simulink model "CellTemp"  (R2017b)
settings: Solver=VariableStepAuto  StartTime=0.0  StopTime=10.0  RelTol=1e-3
undefined symbols (not defined in the file): Battery, Brake, DriveCycle, Driver, g, magnitude, Motor, Sim, TorqueController, TrqSplit, Veh
libraries: simulink x2, AMKMotor x1
settings Model: Creator=Harjot  LastModifiedBy=Harjot

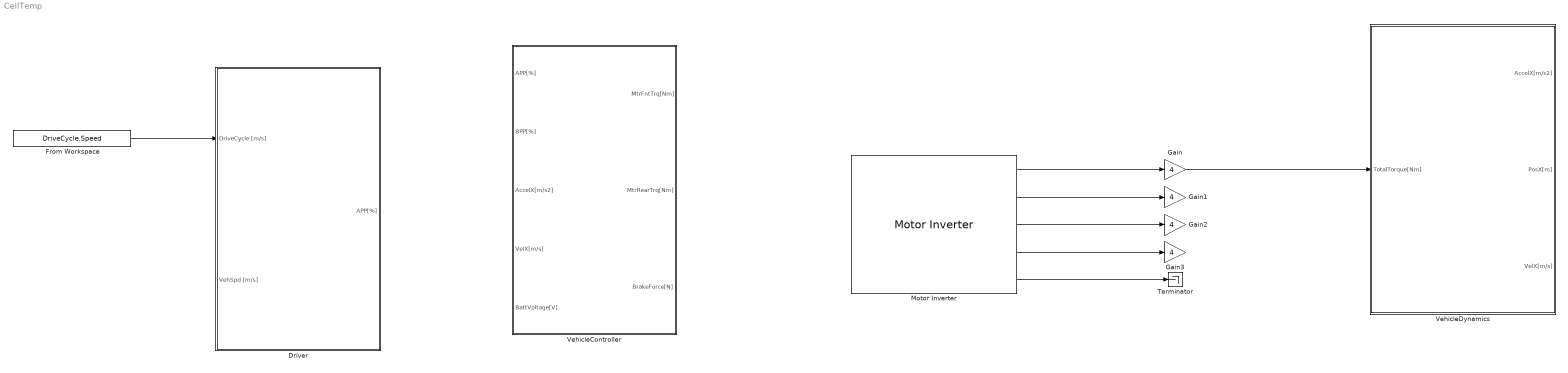
== system CellTemp ==
  Driver : Subsystem
  From Workspace : FromWorkspace  VariableName=DriveCycle.Speed  SampleTime=0
  Gain{,1..3} (4 alike) : Gain  Gain=4
  Motor Inverter : AMKMotor/Motor Inverter
  Terminator : Terminator
  VehicleController : Subsystem  VariantControl=CSMode == 1
  VehicleDynamics : Subsystem
  wires:
  Motor Inverter/1 -> Gain/1
  Gain/1 -> VehicleDynamics/1(TotalTorque[Nm])
  Motor Inverter/2 -> Gain1/1
  Motor Inverter/3 -> Gain2/1
  Motor Inverter/4 -> Gain3/1
  Motor Inverter/5 -> Terminator/1
  From Workspace/1 -> Driver/1(DriveCycle [m/s])

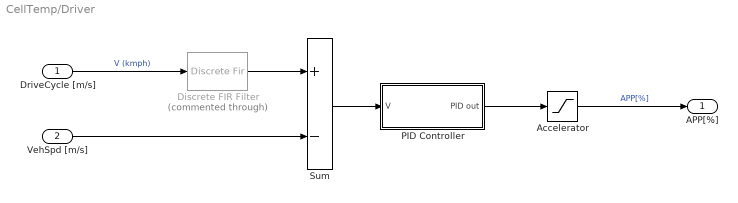
== system CellTemp/Driver ==
  DriveCycle [m/s] : Inport
  VehSpd [m/s] : Inport  Port=2
  Accelerator : Saturate  UpperLimit=100  LowerLimit=0
  Discrete FIR Filter : DiscreteFir  Commented=through  Coefficients=[100:-1:0]/sum([100:-1:0])  SampleTime=Sim.TimeStep
  PID Controller : Subsystem
  Sum : Sum  Inputs=+-
  APP[%] : Outport
  wires:
  VehSpd [m/s]/1 -> Sum/2
  Sum/1 -> PID Controller/1(V)
  DriveCycle [m/s]/1 -> Discrete FIR Filter/1  "V (kmph)"
  PID Controller/1("PID out ") -> Accelerator/1
  Accelerator/1 -> APP[%]/1  "APP[%]"
  Discrete FIR Filter/1 -> Sum/1

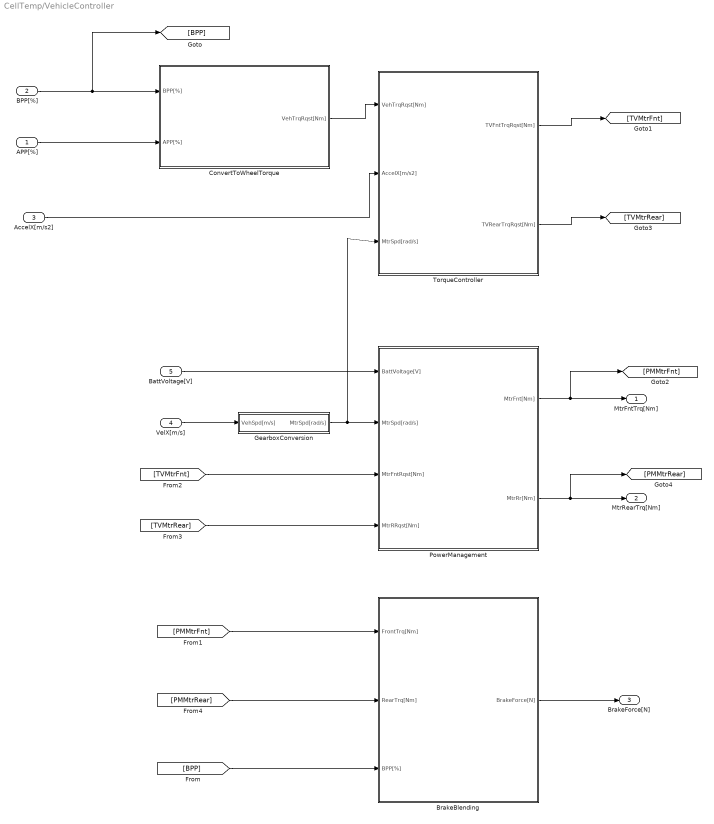
== system CellTemp/VehicleController ==
  APP[%] : Inport
  BPP[%] : Inport  Port=2
  AccelX[m/s2] : Inport  Port=3
  VelX[m/s] : Inport  Port=4
  BattVoltage[V] : Inport  Port=5
  BrakeBlending : Subsystem
  ConvertToWheelTorque : Subsystem
  GearboxConversion : Subsystem
  PowerManagement : Subsystem
  TorqueController : Subsystem
  MtrFntTrq[Nm] : Outport
  MtrRearTrq[Nm] : Outport  Port=2
  BrakeForce[N] : Outport  Port=3
  wires:
  APP[%]/1 -> ConvertToWheelTorque/2(APP[%])
  BPP[%]/1 -> ConvertToWheelTorque/1(BPP[%]), [BPP]
  [PMMtrRear] -> BrakeBlending/2(RearTrq[Nm])
  [PMMtrFnt] -> BrakeBlending/1(FrontTrq[Nm])
  [BPP] -> BrakeBlending/3(BPP[%])
  BrakeBlending/1(BrakeForce[N]) -> BrakeForce[N]/1
  ConvertToWheelTorque/1(VehTrqRqst[Nm]) -> TorqueController/1(VehTrqRqst[Nm])
  GearboxConversion/1(MtrSpd[rad/s]) -> TorqueController/3(MtrSpd[rad/s]), PowerManagement/2(MtrSpd[rad/s])
  VelX[m/s]/1 -> GearboxConversion/1(VehSpd[m/s])
  PowerManagement/2(MtrRr[Nm]) -> MtrRearTrq[Nm]/1, [PMMtrRear]
  PowerManagement/1(MtrFnt[Nm]) -> MtrFntTrq[Nm]/1, [PMMtrFnt]
  [TVMtrRear] -> PowerManagement/4(MtrRRqst[Nm])
  [TVMtrFnt] -> PowerManagement/3(MtrFntRqst[Nm])
  BattVoltage[V]/1 -> PowerManagement/1(BattVoltage[V])
  TorqueController/2(TVRearTrqRqst[Nm]) -> [TVMtrRear]
  TorqueController/1(TVFntTrqRqst[Nm]) -> [TVMtrFnt]
  AccelX[m/s2]/1 -> TorqueController/2(AccelX[m/s2])

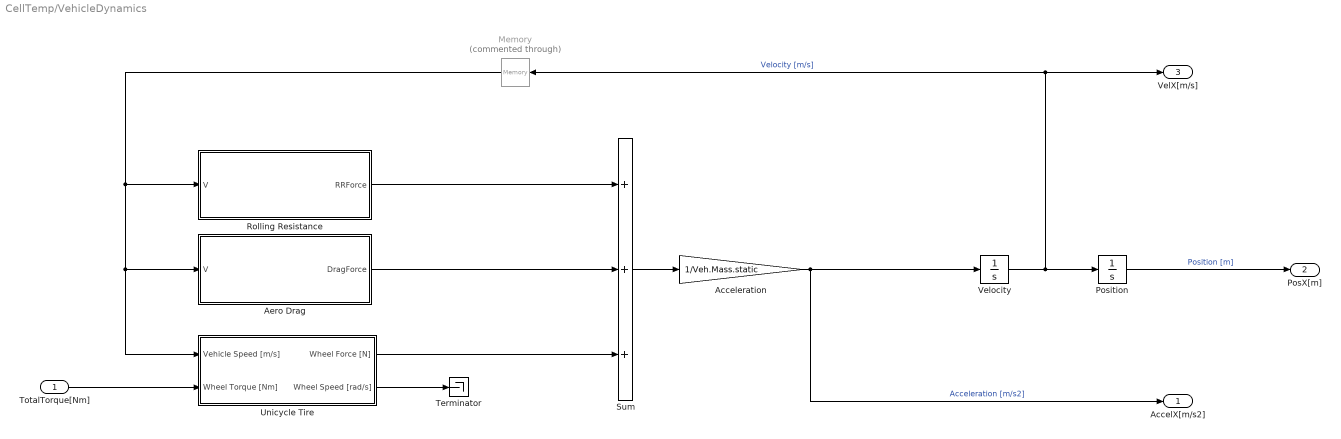
== system CellTemp/VehicleDynamics ==
  TotalTorque[Nm] : Inport
  Acceleration : Gain  Gain=1/Veh.Mass.static
  Aero Drag : Subsystem
  Memory : Memory  Commented=through
  Position : Integrator
  Rolling Resistance : Subsystem
  Sum : Sum  Inputs=+++
  Terminator : Terminator
  Unicycle Tire : Subsystem
  Velocity : Integrator  InitialCondition=DriveCycle.Vi
  AccelX[m/s2] : Outport
  PosX[m] : Outport  Port=2
  VelX[m/s] : Outport  Port=3
  wires:
  Memory/1 -> Unicycle Tire/1(Vehicle Speed [m/s]), Aero Drag/1(V), Rolling Resistance/1(V)
  Acceleration/1 -> AccelX[m/s2]/1, Velocity/1  "Acceleration [m/s2]"
  TotalTorque[Nm]/1 -> Unicycle Tire/2(Wheel Torque [Nm])
  Rolling Resistance/1(RRForce) -> Sum/1
  Aero Drag/1(DragForce) -> Sum/2
  Sum/1 -> Acceleration/1
  Unicycle Tire/1(Wheel Force [N]) -> Sum/3
  Unicycle Tire/2(Wheel Speed [rad/s]) -> Terminator/1
  Velocity/1 -> Memory/1, VelX[m/s]/1, Position/1  "Velocity [m/s]"
  Position/1 -> PosX[m]/1  "Position [m]"

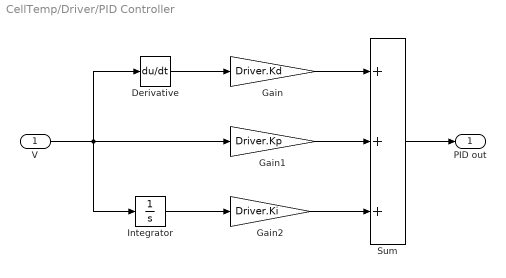
== system CellTemp/Driver/PID Controller ==
  V : Inport
  Derivative : Derivative
  Gain : Gain  Gain=Driver.Kd
  Gain1 : Gain  Gain=Driver.Kp
  Gain2 : Gain  Gain=Driver.Ki
  Integrator : Integrator
  Sum : Sum  Inputs=+++
  "PID out " : Outport
  wires:
  Integrator/1 -> Gain2/1
  V/1 -> Integrator/1, Derivative/1, Gain1/1
  Gain/1 -> Sum/1
  Gain1/1 -> Sum/2
  Gain2/1 -> Sum/3
  Sum/1 -> "PID out "/1
  Derivative/1 -> Gain/1

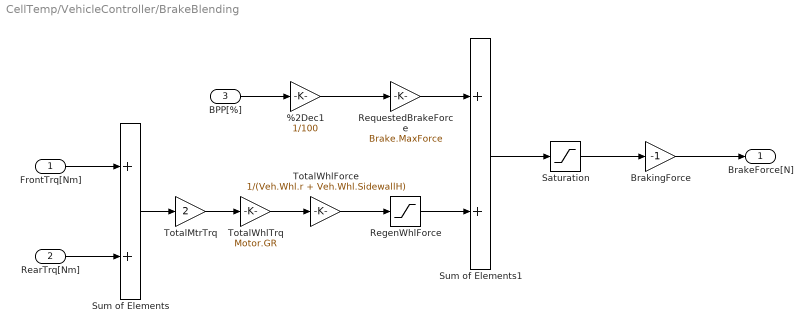
== system CellTemp/VehicleController/BrakeBlending ==
  FrontTrq[Nm] : Inport
  RearTrq[Nm] : Inport  Port=2
  BPP[%] : Inport  Port=3
  %2Dec1 : Gain  Gain=1/100
  BrakingForce : Gain  Gain=-1
  RegenWhlForce : Saturate  UpperLimit=0  LowerLimit=-inf
  RequestedBrakeForce : Gain  Gain=Brake.MaxForce
  Saturation : Saturate  UpperLimit=inf  LowerLimit=0
  Sum of Elements : Sum  Inputs=2
  Sum of Elements1 : Sum
  TotalMtrTrq : Gain  Gain=2
  TotalWhlForce : Gain  Gain=1/(Veh.Whl.r + Veh.Whl.SidewallH)
  TotalWhlTrq : Gain  Gain=Motor.GR
  BrakeForce[N] : Outport
  wires:
  BrakingForce/1 -> BrakeForce[N]/1
  RegenWhlForce/1 -> Sum of Elements1/2
  TotalWhlTrq/1 -> TotalWhlForce/1
  Sum of Elements/1 -> TotalMtrTrq/1
  Saturation/1 -> BrakingForce/1
  Sum of Elements1/1 -> Saturation/1
  TotalWhlForce/1 -> RegenWhlForce/1
  RequestedBrakeForce/1 -> Sum of Elements1/1
  BPP[%]/1 -> %2Dec1/1
  %2Dec1/1 -> RequestedBrakeForce/1
  TotalMtrTrq/1 -> TotalWhlTrq/1
  RearTrq[Nm]/1 -> Sum of Elements/2
  FrontTrq[Nm]/1 -> Sum of Elements/1

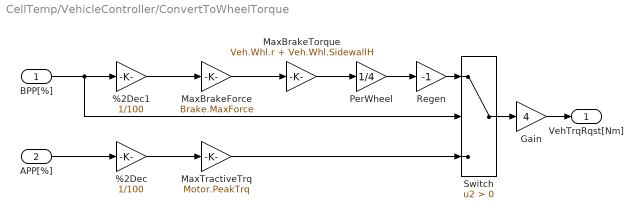
== system CellTemp/VehicleController/ConvertToWheelTorque ==
  BPP[%] : Inport
  APP[%] : Inport  Port=2
  %2Dec : Gain  Gain=1/100
  %2Dec1 : Gain  Gain=1/100
  Gain : Gain  Gain=4
  MaxBrakeForce : Gain  Gain=Brake.MaxForce
  MaxBrakeTorque : Gain  Gain=Veh.Whl.r + Veh.Whl.SidewallH
  "MaxTractiveTrq " : Gain  Gain=Motor.PeakTrq
  PerWheel : Gain  Gain=1/4
  Regen : Gain  Gain=-1
  Switch : Switch  Criteria=u2 > Threshold
  VehTrqRqst[Nm] : Outport
  wires:
  Regen/1 -> Switch/1
  APP[%]/1 -> %2Dec/1
  Switch/1 -> Gain/1
  %2Dec1/1 -> MaxBrakeForce/1
  BPP[%]/1 -> %2Dec1/1, Switch/2
  MaxBrakeTorque/1 -> PerWheel/1
  MaxBrakeForce/1 -> MaxBrakeTorque/1
  %2Dec/1 -> "MaxTractiveTrq "/1
  "MaxTractiveTrq "/1 -> Switch/3
  PerWheel/1 -> Regen/1
  Gain/1 -> VehTrqRqst[Nm]/1

== system CellTemp/VehicleController/GearboxConversion ==
  VehSpd[m/s] : Inport
  MotorGR : Gain  Gain=Motor.GR
  WheelRadius : Gain  Gain=1/(Veh.Whl.r + Veh.Whl.SidewallH)
  MtrSpd[rad/s] : Outport
  wires:
  MotorGR/1 -> MtrSpd[rad/s]/1  "MtrSpd [rad/s]"
  VehSpd[m/s]/1 -> WheelRadius/1
  WheelRadius/1 -> MotorGR/1  "WhlSpd [rad/s]"

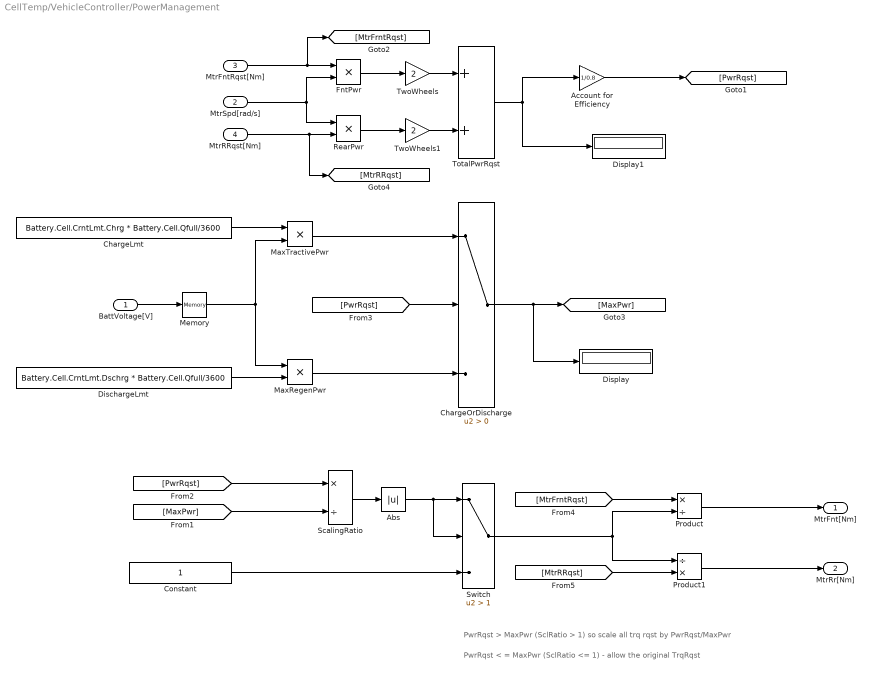
== system CellTemp/VehicleController/PowerManagement ==
  note: PwrRqst < = MaxPwr (SclRatio <= 1) - allow the original TrqRqst
  note: PwrRqst > MaxPwr (SclRatio > 1) so scale all trq rqst by PwrRqst/MaxPwr
  BattVoltage[V] : Inport
  MtrSpd[rad/s] : Inport  Port=2
  MtrFntRqst[Nm] : Inport  Port=3
  MtrRRqst[Nm] : Inport  Port=4
  Abs : Abs
  Account for Efficiency : Gain  Gain=1/0.8
  ChargeLmt : Constant  Value=Battery.Cell.CrntLmt.Chrg * Battery.Cell.Qfull/3600
  ChargeOrDischarge : Switch  Criteria=u2 > Threshold
  Constant : Constant
  DischargeLmt : Constant  Value=Battery.Cell.CrntLmt.Dschrg * Battery.Cell.Qfull/3600
  Display : Display
  Display1 : Display
  FntPwr : Product
  MaxRegenPwr : Product
  MaxTractivePwr : Product
  Memory : Memory  InitialCondition=600
  Product : Product  Inputs=*/
  Product1 : Product  Inputs=/*
  RearPwr : Product
  ScalingRatio : Product  Inputs=*/
  Switch : Switch  Criteria=u2 > Threshold  Threshold=1
  TotalPwrRqst : Sum
  TwoWheels : Gain  Gain=2
  TwoWheels1 : Gain  Gain=2
  MtrFnt[Nm] : Outport
  MtrRr[Nm] : Outport  Port=2
  wires:
  Memory/1 -> MaxRegenPwr/1, MaxTractivePwr/2
  Constant/1 -> Switch/3
  Product1/1 -> MtrRr[Nm]/1
  Product/1 -> MtrFnt[Nm]/1
  [MtrRRqst] -> Product1/2
  [MtrFrntRqst] -> Product/1
  Switch/1 -> Product1/1, Product/2
  MtrFntRqst[Nm]/1 -> FntPwr/1, [MtrFrntRqst]
  [PwrRqst] -> ChargeOrDischarge/2
  TwoWheels/1 -> TotalPwrRqst/1
  TotalPwrRqst/1 -> Account for Efficiency/1, Display1/1
  TwoWheels1/1 -> TotalPwrRqst/2
  RearPwr/1 -> TwoWheels1/1
  FntPwr/1 -> TwoWheels/1
  MtrRRqst[Nm]/1 -> RearPwr/2, [MtrRRqst]
  MtrSpd[rad/s]/1 -> FntPwr/2, RearPwr/1
  Abs/1 -> Switch/2, Switch/1
  ScalingRatio/1 -> Abs/1
  [PwrRqst] -> ScalingRatio/1
  [MaxPwr] -> ScalingRatio/2
  ChargeOrDischarge/1 -> [MaxPwr], Display/1
  MaxRegenPwr/1 -> ChargeOrDischarge/3
  MaxTractivePwr/1 -> ChargeOrDischarge/1
  DischargeLmt/1 -> MaxRegenPwr/2
  BattVoltage[V]/1 -> Memory/1
  ChargeLmt/1 -> MaxTractivePwr/1
  Account for Efficiency/1 -> [PwrRqst]

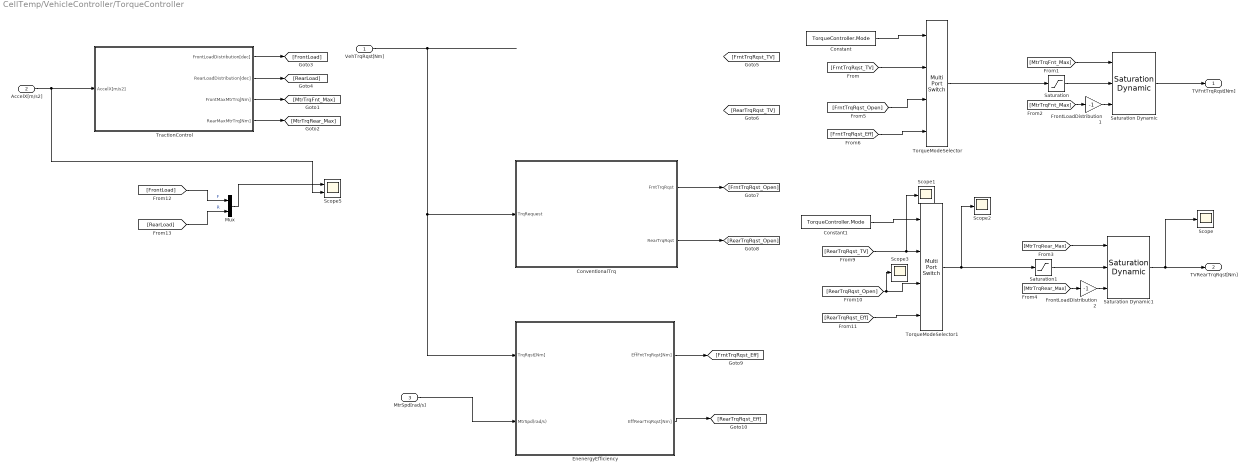
== system CellTemp/VehicleController/TorqueController ==
  VehTrqRqst[Nm] : Inport
  AccelX[m/s2] : Inport  Port=2
  MtrSpd[rad/s] : Inport  Port=3
  Constant : Constant  Value=TorqueController.Mode
  Constant1 : Constant  Value=TorqueController.Mode
  ConventionalTrq : Subsystem
  EnenergyEfficiency : Subsystem
  FrontLoadDistribution1 : Gain  Gain=-1
  FrontLoadDistribution2 : Gain  Gain=-1
  Mux : Mux  Inputs=2
  Saturation : Saturate  UpperLimit=Motor.PeakTrq  LowerLimit=-Motor.PeakTrq
  Saturation Dynamic : simulink/Discontinuities/Saturation Dynamic  OutMin=[]  OutMax=[]  OutDataTypeStr=Inherit: Same as second input  OutDataType=fixdt(1, 16)  OutScaling=2^-10  DoSatur=off
  Saturation Dynamic1 : simulink/Discontinuities/Saturation Dynamic  OutMin=[]  OutMax=[]  OutDataTypeStr=Inherit: Same as second input  OutDataType=fixdt(1, 16)  OutScaling=2^-10  DoSatur=off
  Saturation1 : Saturate  UpperLimit=Motor.PeakTrq  LowerLimit=-Motor.PeakTrq
  Scope{,1..3} (4 alike) : Scope
  Scope5 : Scope  NumInputPorts=2
  TorqueModeSelector : MultiPortSwitch
  TorqueModeSelector1 : MultiPortSwitch
  TractionControl : Subsystem
  TVFntTrqRqst[Nm] : Outport
  TVRearTrqRqst[Nm] : Outport  Port=2
  wires:
  FrontLoadDistribution2/1 -> Saturation Dynamic1/3
  [MtrTrqRear_Max] -> FrontLoadDistribution2/1
  [MtrTrqRear_Max] -> Saturation Dynamic1/1
  Saturation Dynamic1/1 -> Scope/1, TVRearTrqRqst[Nm]/1
  Saturation1/1 -> Saturation Dynamic1/2
  FrontLoadDistribution1/1 -> Saturation Dynamic/3
  [MtrTrqFnt_Max] -> FrontLoadDistribution1/1
  [MtrTrqFnt_Max] -> Saturation Dynamic/1
  Saturation Dynamic/1 -> TVFntTrqRqst[Nm]/1
  Saturation/1 -> Saturation Dynamic/2
  AccelX[m/s2]/1 -> Scope5/2, TractionControl/1(AccelX[m/s2])
  TractionControl/3(FrontMaxMtrTrq[Nm]) -> [MtrTrqFnt_Max]
  TractionControl/4(RearMaxMtrTrq[Nm]) -> [MtrTrqRear_Max]
  TorqueModeSelector/1 -> Saturation/1
  TractionControl/1(FrontLoadDistribution[dec]) -> [FrontLoad]
  TractionControl/2(RearLoadDistribution[dec]) -> [RearLoad]
  ? -> [FrntTrqRqst_TV]
  ? -> [RearTrqRqst_TV]
  VehTrqRqst[Nm]/1 -> EnenergyEfficiency/1(TrqRqst[Nm]), ConventionalTrq/1(TrqRequest)
  ConventionalTrq/1(FrntTrqRqst) -> [FrntTrqRqst_Open]
  ConventionalTrq/2(RearTrqRqst) -> [RearTrqRqst_Open]
  EnenergyEfficiency/1(EffFntTrqRqst[Nm]) -> [FrntTrqRqst_Eff]
  EnenergyEfficiency/2(EffRearTrqRqst[Nm]) -> [RearTrqRqst_Eff]
  TorqueModeSelector1/1 -> Scope2/1, Saturation1/1
  Constant/1 -> TorqueModeSelector/1
  [FrntTrqRqst_TV] -> TorqueModeSelector/2
  [FrntTrqRqst_Open] -> TorqueModeSelector/3
  [FrntTrqRqst_Eff] -> TorqueModeSelector/4
  Constant1/1 -> TorqueModeSelector1/1
  [RearTrqRqst_TV] -> Scope1/1, TorqueModeSelector1/2
  [RearTrqRqst_Open] -> Scope3/1, TorqueModeSelector1/3
  [RearTrqRqst_Eff] -> TorqueModeSelector1/4
  MtrSpd[rad/s]/1 -> EnenergyEfficiency/2(MtrSpd(rad/s))
  Mux/1 -> Scope5/1
  [FrontLoad] -> Mux/1  "F"
  [RearLoad] -> Mux/2  "R"

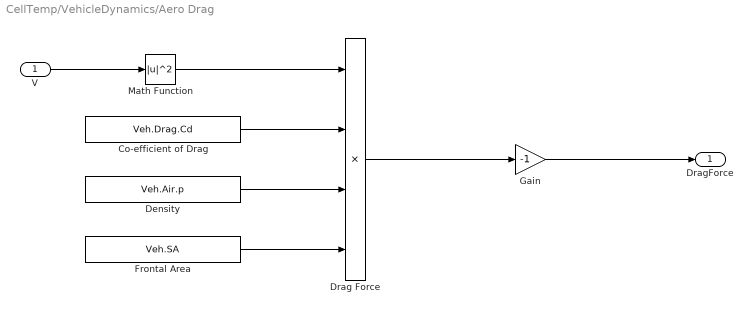
== system CellTemp/VehicleDynamics/Aero Drag ==
  V : Inport
  Co-efficient of Drag : Constant  Value=Veh.Drag.Cd
  Density : Constant  Value=Veh.Air.p
  Drag Force : Product  Inputs=****
  Frontal Area : Constant  Value=Veh.SA
  Gain : Gain  Gain=-1
  Math Function : Math  Operator=magnitude^2  SaturateOnIntegerOverflow=on
  DragForce : Outport
  wires:
  Co-efficient of Drag/1 -> Drag Force/2
  Drag Force/1 -> Gain/1
  V/1 -> Math Function/1
  Math Function/1 -> Drag Force/1
  Density/1 -> Drag Force/3
  Frontal Area/1 -> Drag Force/4
  Gain/1 -> DragForce/1

== system CellTemp/VehicleDynamics/Rolling Resistance ==
  V : Inport
  Coefficient of RR : Lookup_n-D  NumberOfTableDimensions=1  BreakpointsForDimension1=Veh.Tires.rr.Spd  BreakpointsForDimension2=Motor.Efficiency.Spd  Table=Veh.Tires.rr.rr  InternalRulePriority=Speed  RndMeth=Simplest  InputSameDT=on
  Gain : Gain  Gain=-1
  Gain1 : Gain  Gain=g
  Mass : Constant  Value=Veh.Mass.static
  Rolling Resistance : Product
  RRForce : Outport
  wires:
  Rolling Resistance/1 -> Gain/1
  V/1 -> Coefficient of RR/1
  Gain/1 -> RRForce/1
  Coefficient of RR/1 -> Rolling Resistance/1
  Mass/1 -> Gain1/1
  Gain1/1 -> Rolling Resistance/2

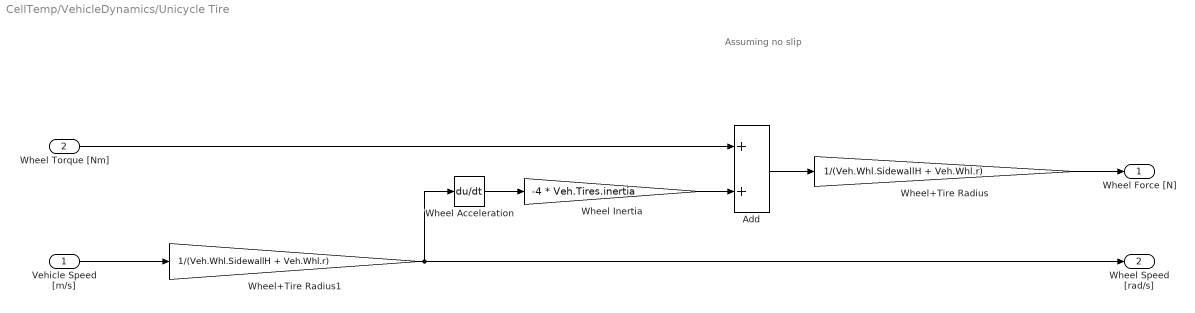
== system CellTemp/VehicleDynamics/Unicycle Tire ==
  note: Assuming no slip
  Vehicle Speed [m/s] : Inport
  Wheel Torque [Nm] : Inport  Port=2
  Add : Sum
  Wheel Acceleration : Derivative
  Wheel Inertia : Gain  Gain=-4 * Veh.Tires.inertia
  Wheel+Tire Radius : Gain  Gain=1/(Veh.Whl.SidewallH + Veh.Whl.r)
  Wheel+Tire Radius1 : Gain  Gain=1/(Veh.Whl.SidewallH + Veh.Whl.r)
  Wheel Force [N] : Outport
  Wheel Speed [rad/s] : Outport  Port=2
  wires:
  Wheel+Tire Radius/1 -> Wheel Force [N]/1
  Vehicle Speed [m/s]/1 -> Wheel+Tire Radius1/1
  Wheel+Tire Radius1/1 -> Wheel Speed [rad/s]/1, Wheel Acceleration/1
  Wheel Acceleration/1 -> Wheel Inertia/1
  Add/1 -> Wheel+Tire Radius/1
  Wheel Torque [Nm]/1 -> Add/1
  Wheel Inertia/1 -> Add/2

== system CellTemp/VehicleController/TorqueController/ConventionalTrq ==
  TrqRequest : Inport
  WhlTrqRqst : Gain  Gain=1/4
  FrntTrqRqst : Outport
  RearTrqRqst : Outport  Port=2
  wires:
  TrqRequest/1 -> WhlTrqRqst/1
  WhlTrqRqst/1 -> RearTrqRqst/1, FrntTrqRqst/1

== system CellTemp/VehicleController/TorqueController/EnenergyEfficiency ==
  TrqRqst[Nm] : Inport
  MtrSpd(rad/s) : Inport  Port=2
  FrontMtrTrq : Lookup_n-D  BreakpointsForDimension1=TrqSplit.Spd  BreakpointsForDimension2=TrqSplit.Trq  Table=TrqSplit.FrontTrq  InternalRulePriority=Speed  RndMeth=Simplest  InputSameDT=on
  RearMtrTrq : Lookup_n-D  BreakpointsForDimension1=TrqSplit.Spd  BreakpointsForDimension2=TrqSplit.Trq  Table=TrqSplit.RearTrq  InternalRulePriority=Speed  RndMeth=Simplest  InputSameDT=on
  EffFntTrqRqst[Nm] : Outport
  EffRearTrqRqst[Nm] : Outport  Port=2
  wires:
  FrontMtrTrq/1 -> EffFntTrqRqst[Nm]/1
  RearMtrTrq/1 -> EffRearTrqRqst[Nm]/1
  MtrSpd(rad/s)/1 -> RearMtrTrq/1, FrontMtrTrq/1
  TrqRqst[Nm]/1 -> FrontMtrTrq/2, RearMtrTrq/2

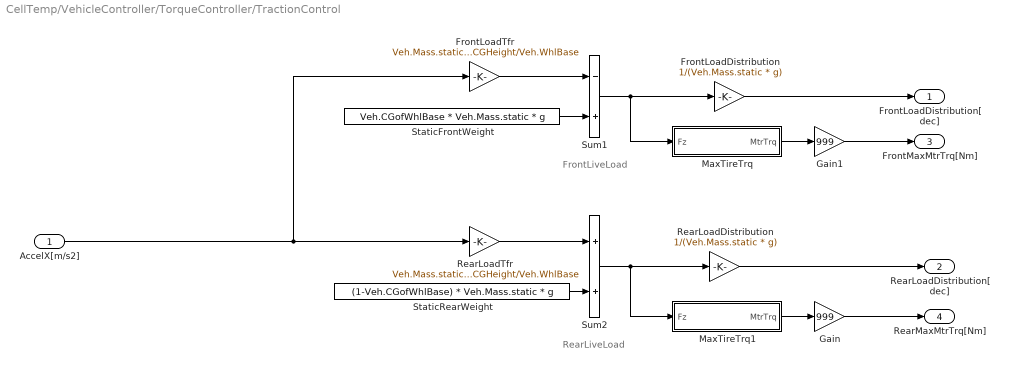
== system CellTemp/VehicleController/TorqueController/TractionControl ==
  note: FrontLiveLoad
  note: RearLiveLoad
  AccelX[m/s2] : Inport
  FrontLoadDistribution : Gain  Gain=1/(Veh.Mass.static * g)
  FrontLoadTfr : Gain  Gain=Veh.Mass.static*Veh.CGHeight/Veh.WhlBase
  Gain : Gain  Gain=999
  Gain1 : Gain  Gain=999
  MaxTireTrq : Subsystem
  MaxTireTrq1 : Subsystem
  RearLoadDistribution : Gain  Gain=1/(Veh.Mass.static * g)
  RearLoadTfr : Gain  Gain=Veh.Mass.static*Veh.CGHeight/Veh.WhlBase
  StaticFrontWeight : Constant  Value=Veh.CGofWhlBase * Veh.Mass.static * g
  StaticRearWeight : Constant  Value=(1-Veh.CGofWhlBase) * Veh.Mass.static * g
  Sum1 : Sum  Inputs=-+
  Sum2 : Sum
  FrontLoadDistribution[dec] : Outport
  RearLoadDistribution[dec] : Outport  Port=2
  FrontMaxMtrTrq[Nm] : Outport  Port=3
  RearMaxMtrTrq[Nm] : Outport  Port=4
  wires:
  MaxTireTrq1/1(MtrTrq) -> Gain/1
  MaxTireTrq/1(MtrTrq) -> Gain1/1
  RearLoadDistribution/1 -> RearLoadDistribution[dec]/1
  FrontLoadTfr/1 -> Sum1/1
  RearLoadTfr/1 -> Sum2/1
  StaticRearWeight/1 -> Sum2/2
  Sum1/1 -> FrontLoadDistribution/1, MaxTireTrq/1(Fz)
  Sum2/1 -> RearLoadDistribution/1, MaxTireTrq1/1(Fz)
  StaticFrontWeight/1 -> Sum1/2
  FrontLoadDistribution/1 -> FrontLoadDistribution[dec]/1
  AccelX[m/s2]/1 -> FrontLoadTfr/1, RearLoadTfr/1
  Gain/1 -> RearMaxMtrTrq[Nm]/1
  Gain1/1 -> FrontMaxMtrTrq[Nm]/1

== system CellTemp/VehicleController/TorqueController/TractionControl/MaxTireTrq ==
  Fz : Inport
  MaxMtrTorque : Gain  Gain=1/Motor.GR
  MaxTireForce : Gain  Gain=Veh.Tires.Ks
  MaxWhlTorque : Gain  Gain=Veh.Whl.r + Veh.Whl.SidewallH
  SplitAxle : Gain  Gain=1/2
  MtrTrq : Outport
  wires:
  MaxMtrTorque/1 -> MtrTrq/1
  SplitAxle/1 -> MaxTireForce/1
  MaxWhlTorque/1 -> MaxMtrTorque/1
  Fz/1 -> SplitAxle/1
  MaxTireForce/1 -> MaxWhlTorque/1

== system CellTemp/VehicleController/TorqueController/TractionControl/MaxTireTrq1 ==
  Fz : Inport
  MaxMtrTorque : Gain  Gain=1/Motor.GR
  MaxTireForce : Gain  Gain=Veh.Tires.Ks
  MaxWhlTorque : Gain  Gain=Veh.Whl.r + Veh.Whl.SidewallH
  SplitAxle : Gain  Gain=1/2
  MtrTrq : Outport
  wires:
  MaxMtrTorque/1 -> MtrTrq/1
  SplitAxle/1 -> MaxTireForce/1
  MaxWhlTorque/1 -> MaxMtrTorque/1
  Fz/1 -> SplitAxle/1
  MaxTireForce/1 -> MaxWhlTorque/1
